simulink model "UZ_EnDat_be4_diffrework"  (R2023b)
settings: Solver=FixedStepDiscrete  StartTime=0  StopTime=0.002  RelTol=1e-3
model workspace (MAT data in the model file):
  Select = 0
libraries: hdlsllib x207, simulink x17, simulink_extras x3
(part 1 of 5)
settings Model: DataTypeOverride=Off  SimulationMode=accelerator  NumberOfSteps=10  PacingRate=1000  Creator=ELSYS_PC  LastModifiedBy=ELSYS_PC
settings SolverCC: AlgebraicLoopSolver=TrustRegion
settings DataIOCC: LimitDataPoints=on  SaveOutput=off  SaveTime=off
settings OptimizationCC: BlockReduction=off  ConditionallyExecuteInputs=off  DefaultParameterBehavior=Inlined  InheritOutputTypeSmallerThanSingle=on  LifeSpan=inf
settings DebuggingCC: AlgebraicLoopMsg=error  SingleTaskRateTransMsg=error  UnconnectedInputMsg=warning  UnconnectedOutputMsg=warning  UnconnectedLineMsg=warning  AllowSymbolicDim=off  StrictBusMsg=ErrorOnBusTreatedAsVector  SFUnexpectedBacktrackingDiag=warning  SFNoUnconditionalDefaultTransitionDiag=warning  SFExecutionAtInitializationDiag=none  ArithmeticOperatorsInVariantConditions=warning
settings HardwareCC: ProdBitPerPointer=32  ProdBitPerSizeT=32  ProdBitPerPtrDiffT=32  ProdLargestAtomicFloat=None  ProdIntDivRoundTo=Undefined  ProdEndianess=Unspecified  ProdWordSize=32  ProdHWDeviceType=ASIC/FPGA->ASIC/FPGA  TargetBitPerPointer=64  TargetBitPerSizeT=64  TargetBitPerPtrDiffT=64  TargetLongLongMode=on  TargetIntDivRoundTo=Zero  TargetEndianess=LittleEndian  TargetWordSize=64  TargetHWDeviceType=Custom Processor->MATLAB Host Computer  ProdEqTarget=off
settings ModelReferenceCC: EnableRefExpFcnMdlSchedulingChecks=on
settings SFSimCC: SimUseLocalCustomCode=off  CustomCodeUndefinedFunction=UseInterfaceOnly
settings RTWCC: RTWUseLocalCustomCode=off
settings CodeAppCC: StateflowObjectComments=on
settings GRTTargetCC: TargetLangStandard=C89/C90 (ANSI)  RTWCAPISignals=on  RTWCAPIParams=on
settings ConfigComp: CovScope=ReferencedModels  CovMetricSettings=dw  CovSaveCumulativeToWorkspaceVar=on  CovSaveSingleToWorkspaceVar=on  CovExternalEMLEnable=off  CovSFcnEnable=off  DVTestSuiteOptimization=Auto  DVDetectOutOfBounds=on  DVModelReferenceHarness=on  DVHarnessSource=Signal Editor  DVRebuildModelRepresentation=IfChangeIsDetected

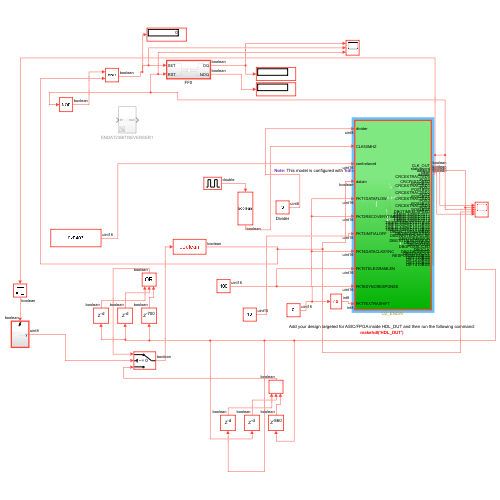
[thumbnail: Simulink's stored preview of the top-level diagram]
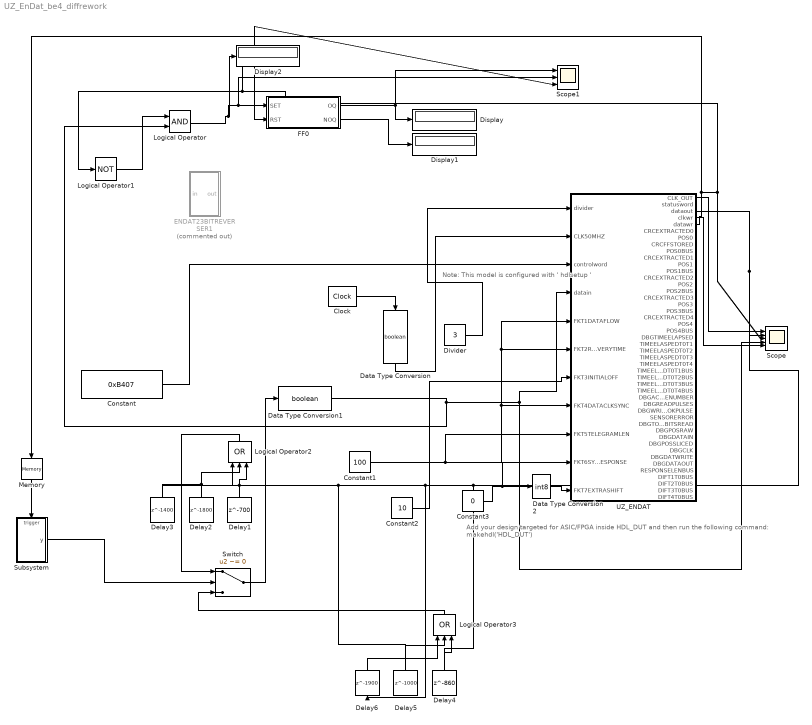
== system UZ_EnDat_be4_diffrework ==
  note: Note: This model is configured with ' hdlsetup '
  note: Add your design targeted for ASIC/FPGA inside HDL_DUT and then run the following command:
      | makehdl('HDL_DUT')
  Clock : simulink_extras/Flip Flops/Clock  period=2E-8
  Constant : Constant  Value=0xB407  OutDataTypeStr=uint16  SampleTime=-1
  Constant1 : Constant  Value=100  OutDataTypeStr=uint16  SampleTime=-1
  Constant2 : Constant  Value=10  OutDataTypeStr=uint16  SampleTime=-1
  Constant3 : Constant  Value=0  OutDataTypeStr=uint16  SampleTime=-1
  Data Type Conversion : DataTypeConversion  OutDataTypeStr=boolean  SaturateOnIntegerOverflow=off  RndMeth=Floor
  Data Type Conversion1 : DataTypeConversion  OutDataTypeStr=boolean  SaturateOnIntegerOverflow=off  RndMeth=Floor
  Data Type Conversion2 : DataTypeConversion  OutDataTypeStr=int8  SaturateOnIntegerOverflow=off  RndMeth=Floor
  Delay1 : Delay  DelayLength=700
  Delay2 : Delay  DelayLength=1800
  Delay3 : Delay  DelayLength=1400
  Delay4 : Delay  DelayLength=860
  Delay5 : Delay  DelayLength=1000
  Delay6 : Delay  DelayLength=1900
  Display : Display
  Display1 : Display
  Display2 : Display
  Divider : Constant  Value=3  OutMin=0  OutMax=7  OutDataTypeStr=uint8  SampleTime=-1
  ENDAT23BITREVERSER1 : Subsystem  Commented=on
  FF0 : Subsystem  TreatAsAtomicUnit=on
      settings: LibrarySourceBlock=|
      | hdlsllib/Ports &
      | Subsystems/Triggered
      | Subsystem
  Logical Operator : Logic  AllPortsSameDT=off  OutDataTypeStr=boolean
  Logical Operator1 : Logic  Operator=NOT  AllPortsSameDT=off  OutDataTypeStr=boolean
  Logical Operator2 : Logic  Operator=OR  Inputs=3  AllPortsSameDT=off  OutDataTypeStr=boolean
  Logical Operator3 : Logic  Operator=OR  Inputs=3  AllPortsSameDT=off  OutDataTypeStr=boolean
  Memory : Memory  InheritSampleTime=on
  Scope : Scope  NumInputPorts=5
  Scope1 : Scope  NumInputPorts=3
  Subsystem : Subsystem
  Switch : Switch  Criteria=u2 ~= 0  SaturateOnIntegerOverflow=off  InputSameDT=off
  UZ_ENDAT : Subsystem  TreatAsAtomicUnit=on
  wires:
  Constant/1 -> UZ_ENDAT/3(controlword)
  Data Type Conversion/1 -> UZ_ENDAT/2(CLK50MHZ)
  Divider/1 -> UZ_ENDAT/1(divider)
  Clock/1 -> Data Type Conversion/1
  Data Type Conversion1/1 -> Logical Operator/2, Scope/4, UZ_ENDAT/4(datain)
  Delay1/1 -> Logical Operator2/3
  UZ_ENDAT/1(CLK_OUT) -> Scope/1
  UZ_ENDAT/5(datawr) -> Memory/1, Scope1/3, FF0/2(RST), Logical Operator1/1, Scope/3
  Constant1/1 -> UZ_ENDAT/5(FKT1DATAFLOW), UZ_ENDAT/6(FKT2RECOVERYTIME), UZ_ENDAT/8(FKT4DATACLKSYNC), UZ_ENDAT/9(FKT5TELEGRAMLEN)
  Constant2/1 -> UZ_ENDAT/7(FKT3INITIALOFF)
  FF0/1(OQ) -> Scope1/1, Display/1
  Logical Operator/1 -> Scope1/2, FF0/1(SET), Display2/1
  FF0/2(NOQ) -> Display1/1
  Logical Operator1/1 -> Logical Operator/1
  Delay2/1 -> Logical Operator2/2
  Delay3/1 -> Logical Operator2/1
  Logical Operator2/1 -> Switch/1
  Switch/1 -> Data Type Conversion1/1
  Delay6/1 -> Logical Operator3/1
  Delay5/1 -> Logical Operator3/2
  Logical Operator3/1 -> Switch/3
  Delay4/1 -> Logical Operator3/3
  UZ_ENDAT/3(dataout) -> Delay4/1, Delay6/1, Delay3/1, Delay2/1, Delay1/1, Delay5/1, Scope/2
  Subsystem/1(y) -> Switch/2
  Memory/1 -> Subsystem/Trigger
  UZ_ENDAT/4(clkwr) -> Scope/5
  Constant3/1 -> UZ_ENDAT/10(FKT6SYNCRESPONSE), Data Type Conversion2/1
  Data Type Conversion2/1 -> UZ_ENDAT/11(FKT7EXTRASHIFT)

== system UZ_EnDat_be4_diffrework/ENDAT23BITREVERSER1 ==
  in : Inport
  16BITREVERSER : Subsystem
  16BITREVERSER1 : Subsystem
  Bit Concat : hdlsllib/Logic and Bit Operations/Bit Concat  numInputs=2
  Bit Shift : hdlsllib/Logic and Bit Operations/Bit Shift  mode=Shift Right Logical  N=8
  Bit Slice : hdlsllib/Logic and Bit Operations/Bit Slice  lidx=15  ridx=0
  Bit Slice1 : hdlsllib/Logic and Bit Operations/Bit Slice  lidx=22  ridx=16
  out : Outport
  wires:
  Bit Concat/1 -> Bit Shift/1
  Bit Shift/1 -> out/1
  in/1 -> Bit Slice1/1, Bit Slice/1
  Bit Slice/1 -> 16BITREVERSER/1(in)
  Bit Slice1/1 -> 16BITREVERSER1/1(in)
  16BITREVERSER/1(out) -> Bit Concat/1
  16BITREVERSER1/1(out) -> Bit Concat/2

== system UZ_EnDat_be4_diffrework/FF0 ==
  SET : Inport
  RST : Inport  Port=2
  S-R Flip-Flop : simulink_extras/Flip Flops/S-R Flip-Flop  initial_condition=0
  OQ : Outport
  NOQ : Outport  Port=2
  wires:
  SET/1 -> S-R Flip-Flop/1
  RST/1 -> S-R Flip-Flop/2
  S-R Flip-Flop/1 -> OQ/1
  S-R Flip-Flop/2 -> NOQ/1

== system UZ_EnDat_be4_diffrework/Subsystem ==
  Trigger : TriggerPort  VariantControl=(inherit)  PortDimensions=1
  Counter Limited : hdlsllib/Sources/Counter Limited  uplimit=1  tsamp=-1
  y : Outport
  wires:
  Counter Limited/1 -> y/1

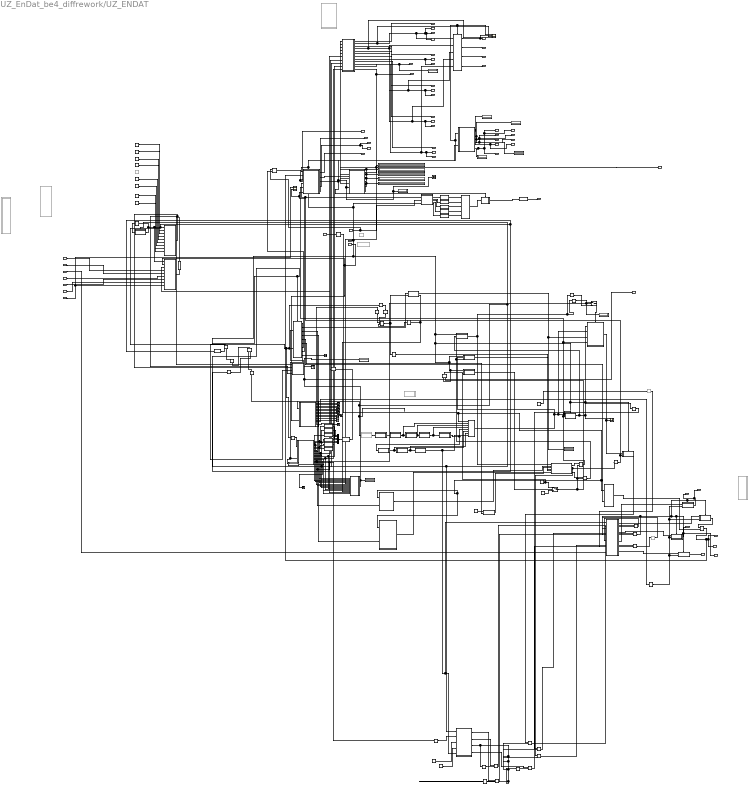
== system UZ_EnDat_be4_diffrework/UZ_ENDAT ==
  note: 0=12.5;1=6,25;2=3,125;3=1,5625
  divider : Inport  OutDataTypeStr=uint8  SampleTime=1e-8
  CLK50MHZ : Inport  Port=2  SampleTime=1e-8
  controlword : Inport  Port=3  OutDataTypeStr=uint16  SampleTime=1e-8
  datain : Inport  Port=4  OutDataTypeStr=boolean  SampleTime=1e-8
  FKT1DATAFLOW : Inport  Port=5  OutDataTypeStr=uint16  SampleTime=1e-8
  FKT2RECOVERYTIME : Inport  Port=6  OutDataTypeStr=uint16  SampleTime=1e-8
  FKT3INITIALOFF : Inport  Port=7  OutDataTypeStr=uint16  SampleTime=1e-8
  FKT4DATACLKSYNC : Inport  Port=8  OutDataTypeStr=uint16  SampleTime=1e-8
  FKT5TELEGRAMLEN : Inport  Port=9  OutDataTypeStr=uint16  SampleTime=1e-8
  FKT6SYNCRESPONSE : Inport  Port=10  OutDataTypeStr=uint16  SampleTime=1e-8
  FKT7EXTRASHIFT : Inport  Port=11  OutDataTypeStr=int8  SampleTime=1e-8
  16BIT_SPLITTER1 : Subsystem  Commented=on  TreatAsAtomicUnit=on
  16bitgather : Subsystem
      settings: LibrarySourceBlock=|
      | hdlsllib/Ports &
      | Subsystems/Subsystem
  2CLKDELAY : Delay  DelayLengthSource=Input port  DelayLength=10  DelayLengthUpperLimit=127  PreventDirectFeedthrough=on
      settings: InputPortMap=u0,p1
  5timestorage : Subsystem
      settings: LibrarySourceBlock=|
      | hdlsllib/Ports &
      | Subsystems/Subsystem
  8BIT_SPLITTER : Subsystem  TreatAsAtomicUnit=on
  8BIT_SPLITTER1 : Subsystem  TreatAsAtomicUnit=on
  Bits to Word : hdlsllib/Logic and Bit Operations/Bits to Word
  CLKCNTER_ACT : Subsystem
      settings: LibrarySourceBlock=|
      | hdlsllib/Ports &
      | Subsystems/Subsystem
  CLKCNTER_NOSTOP : Subsystem
      settings: LibrarySourceBlock=|
      | hdlsllib/Ports &
      | Subsystems/Subsystem
  CLKCNTER_RAMPUP : Subsystem
      settings: LibrarySourceBlock=|
      | hdlsllib/Ports &
      | Subsystems/Subsystem
  CLKDIV1 : Subsystem
  CLKDIV2 : Subsystem  Commented=through
  CLKDIV3 : Subsystem
  CLKDIV4 : Subsystem
  CLKDIV5 : Subsystem
  CLKDIV6 : Subsystem
  CLKDIV7 : Subsystem
  CLKDIV8 : Subsystem
  CLKDIV9 : Subsystem
  CONTROLWORDRAW : Subsystem
      settings: LibrarySourceBlock=|
      | hdlsllib/Ports &
      | Subsystems/Subsystem
  CONTROLWORDSTORED : Subsystem
      settings: LibrarySourceBlock=|
      | hdlsllib/Ports &
      | Subsystems/Subsystem
  CRC_Check : Subsystem  TreatAsAtomicUnit=on
  Compare To Constant : hdlsllib/Logic and Bit Operations/Compare To Constant  relop===  const=1  OutDataTypeStr=boolean
  Compare To Constant1 : hdlsllib/Logic and Bit Operations/Compare To Constant  relop===  const=1  OutDataTypeStr=boolean
  Compare To Constant2 : hdlsllib/Logic and Bit Operations/Compare To Constant  relop===  const=0  OutDataTypeStr=boolean
  Compare To Constant3 : hdlsllib/Logic and Bit Operations/Compare To Constant  relop=>=  const=3  OutDataTypeStr=boolean
  Compare To Constant4 : hdlsllib/Logic and Bit Operations/Compare To Constant  relop=>=  const=2  OutDataTypeStr=boolean
  Constant10 : Constant  Commented=on  Value=3  OutDataTypeStr=fixdt(0,4,0)  SampleTime=-1
  Constant11 : Constant  Commented=on  Value=0xB407  OutDataTypeStr=uint16  SampleTime=-1
  Constant12 : Constant  Value=48  OutDataTypeStr=uint16  SampleTime=-1
  Constant13 : Constant  Value=8  OutDataTypeStr=uint8  SampleTime=-1
  Constant3 : Constant  OutDataTypeStr=boolean  SampleTime=-1
  Constant6 : Constant  Value=51  OutDataTypeStr=uint16  SampleTime=-1
  ControlWordRAM : Constant  Value=0  VectorParams1D=off  OutDataTypeStr=uint8  SampleTime=-1
  DATA2CLOCKSYNCER : Subsystem
  DATA2CLOCKSYNCER1 : Subsystem  Commented=on
  DATAFLOWCHGER : Subsystem
  Data Type Conversion : DataTypeConversion  OutDataTypeStr=fixdt(0,4,0)  RndMeth=Nearest
  Data Type Conversion1 : DataTypeConversion  OutDataTypeStr=uint8  SaturateOnIntegerOverflow=off  RndMeth=Floor
  Data Type Conversion{2..12} (11 alike) : DataTypeConversion  OutMax=1  OutDataTypeStr=fixdt(0,1)  SaturateOnIntegerOverflow=off  RndMeth=Floor
  Delay : Delay  DelayLength=10  InitialCondition=0
  Delay1 : Delay  DelayLengthSource=Input port  DelayLengthUpperLimit=127  InitialCondition=0
      settings: InputPortMap=u0,p1
  Delay2 : Delay  DelayLength=1
  Delay3 : Delay  DelayLength=1
  Delay4 : Delay  DelayLength=0
  Detect Change : simulink/Logic and Bit Operations/Detect Change  vinit=0  OutDataTypeStr=boolean
      settings: LibrarySourceBlock=|
      | hdlsllib/Logic and Bit
      | Operations/Detect
      | Change
  Display{,1..15} (16 alike) : Display
      Display settings: Format=hex (Stored Integer)
      Display1 settings: Format=binary (Stored Integer)
      Display2 settings: Format=binary (Stored Integer)
      Display3 settings: Format=binary (Stored Integer)
      Display4 settings: Format=binary (Stored Integer)
      Display5 settings: Format=binary (Stored Integer)
      Display7 settings: Format=hex (Stored Integer)
      Display8 settings: Format=hex (Stored Integer)
      Display9 settings: Format=hex (Stored Integer)
  Dual Port RAM System : hdlsllib/HDL RAMs/Dual Port RAM System  RAMType=Dual port  AsyncRead=off  WriteOutputValue=New data  RAMInitialValue=0  allowBusInputs=off  WritesHaveOutput=on  NumReads=0  NumWrites=1  SimulateUsing=Code generation
  EndatControlRAM : Constant  VectorParams1D=off  OutDataTypeStr=uint8  SampleTime=-1
  FKT1 : Constant  Value=2  VectorParams1D=off  OutDataTypeStr=uint8  SampleTime=-1
  FKT2 : Constant  Value=3  VectorParams1D=off  OutDataTypeStr=uint8  SampleTime=-1
  FKT3 : Constant  Commented=on  Value=4  VectorParams1D=off  OutDataTypeStr=uint8  SampleTime=-1
  FKT4 : Constant  Value=5  VectorParams1D=off  OutDataTypeStr=uint8  SampleTime=-1
  FKT5 : Constant  Value=6  VectorParams1D=off  OutDataTypeStr=uint8  SampleTime=-1
  FKT6 : Constant  Value=7  VectorParams1D=off  OutDataTypeStr=uint8  SampleTime=-1
  FKT7 : Constant  Value=8  VectorParams1D=off  OutDataTypeStr=uint8  SampleTime=-1
  INITIALOFF : Subsystem
  Logical Operator{,1,7,9,13..14,16,18,20} (9 alike) : Logic  AllPortsSameDT=off  OutDataTypeStr=boolean
  Logical Operator10 : Logic  Operator=NOT  Inputs=3  AllPortsSameDT=off  OutDataTypeStr=boolean
  Logical Operator{5,11,15,22..23} (5 alike) : Logic  Operator=OR  AllPortsSameDT=off  OutDataTypeStr=boolean
  Logical Operator{2..4,17,19,21,24,27} (8 alike) : Logic  Operator=NOT  AllPortsSameDT=off  OutDataTypeStr=boolean
  Logical Operator25 : Logic  Commented=through  Operator=NOT  AllPortsSameDT=off  OutDataTypeStr=boolean
  Logical Operator26 : Logic  Commented=through  Operator=NOT  AllPortsSameDT=off  OutDataTypeStr=boolean
  Logical Operator6 : Logic  Operator=NOT  Inputs=3  AllPortsSameDT=off  OutDataTypeStr=boolean
  Logical Operator8 : Logic  Inputs=3  AllPortsSameDT=off  OutDataTypeStr=boolean
  ManualSerialize : Subsystem
      settings: LibrarySourceBlock=|
      | hdlsllib/Ports &
      | Subsystems/Subsystem
  Memory : Memory  InheritSampleTime=on
  Multiport Switch : MultiPortSwitch  DataPortOrder=Zero-based contiguous  Inputs=7  DataPortIndices={8,16,32,64}  zeroidx=on  SaturateOnIntegerOverflow=off  InputSameDT=off
  OUTPUTCONTROLCONTINIOUS : Subsystem
      settings: LibrarySourceBlock=|
      | hdlsllib/Ports &
      | Subsystems/Subsystem
  RAM_SELECTOR : MultiPortSwitch  DataPortOrder=Zero-based contiguous  Inputs=8  DataPortForDefault=Additional data port  zeroidx=on  OutDataTypeStr=uint8  SaturateOnIntegerOverflow=off  InputSameDT=off
  RAM_SELECTOR1 : MultiPortSwitch  DataPortOrder=Zero-based contiguous  Inputs=8  DataPortForDefault=Additional data port  zeroidx=on  SaturateOnIntegerOverflow=off  InputSameDT=off
  RAM_SELECTOR2 : MultiPortSwitch  Commented=on  DataPortOrder=Zero-based contiguous  Inputs=16  DataPortForDefault=Additional data port  zeroidx=on  SaturateOnIntegerOverflow=off  InputSameDT=off
  RECOVERYTIMESELECTOR : Subsystem
  RESPONSESLICER5X : Subsystem
  Scope : Scope
  Scope1 : Scope  NumInputPorts=2
  Scope2 : Scope  NumInputPorts=2
  Scope3 : Scope  NumInputPorts=4
  SetZero32modified : Subsystem  Commented=on
  SetZeroBool : Subsystem
  SetZeroBool1 : Subsystem
  SetZeroBool2 : Subsystem
  SetZeroBool3 : Subsystem
  SetZeroBool4 : Subsystem
  SetZeroBool5 : Subsystem
  Signal Specification : SignalSpecification  OutDataTypeStr=uint16
  Storage16 : Subsystem
      settings: LibrarySourceBlock=|
      | hdlsllib/Ports &
      | Subsystems/Subsystem
  Subsystem : Subsystem
  Subsystem1 : Subsystem
  Subsystem2 : Subsystem
  Subsystem6 : Subsystem
  Switch : Switch  Criteria=u2 > Threshold  SaturateOnIntegerOverflow=off  InputSameDT=off
  Terminator{,1,4,12..17,19..25} (16 alike) : Terminator
  Vector Concatenate : Concatenate  NumInputs=6
  Vector Concatenate1 : Concatenate  NumInputs=5
  deadtime : Switch  Threshold=2000  SaturateOnIntegerOverflow=off  InputSameDT=off
  deadtimeconst1 : Constant  OutDataTypeStr=boolean  SampleTime=-1
  deadtimeconst2 : Constant  Value=0  OutDataTypeStr=boolean  SampleTime=-1
  ramselektor : Subsystem  TreatAsAtomicUnit=on
      settings: LibrarySourceBlock=|
      | hdlsllib/Ports &
      | Subsystems/Triggered
      | Subsystem
  responseslicer5 : Subsystem  Commented=on  TreatAsAtomicUnit=on
      settings: LibrarySourceBlock=|
      | hdlsllib/Ports &
      | Subsystems/Subsystem
  timingprovider : Subsystem
      settings: LibrarySourceBlock=|
      | hdlsllib/Ports &
      | Subsystems/Subsystem
  CLK_OUT : Outport  VectorParamsAs1DForOutWhenUnconnected=off
  statusword : Outport  Port=2  OutDataTypeStr=uint16  VectorParamsAs1DForOutWhenUnconnected=off
  dataout : Outport  Port=3  OutDataTypeStr=boolean  VectorParamsAs1DForOutWhenUnconnected=off
  clkwr : Outport  Port=4  OutDataTypeStr=boolean  VectorParamsAs1DForOutWhenUnconnected=off
  datawr : Outport  Port=5  OutDataTypeStr=boolean  VectorParamsAs1DForOutWhenUnconnected=off
  CRCEXTRACTED0 : Outport  Port=6  OutDataTypeStr=uint8  VectorParamsAs1DForOutWhenUnconnected=off
  POS0 : Outport  Port=7  OutDataTypeStr=uint32  VectorParamsAs1DForOutWhenUnconnected=off
  CRCFFSTORED : Outport  Port=8  OutDataTypeStr=uint8  VectorParamsAs1DForOutWhenUnconnected=off
  POS0BUS : Outport  Port=9  OutDataTypeStr=uint32  VectorParamsAs1DForOutWhenUnconnected=off
  CRCEXTRACTED1 : Outport  Port=10  OutDataTypeStr=uint8  VectorParamsAs1DForOutWhenUnconnected=off
  POS1 : Outport  Port=11  OutDataTypeStr=uint32  VectorParamsAs1DForOutWhenUnconnected=off
  POS1BUS : Outport  Port=12  OutDataTypeStr=uint32  VectorParamsAs1DForOutWhenUnconnected=off
  CRCEXTRACTED2 : Outport  Port=13  OutDataTypeStr=uint8  VectorParamsAs1DForOutWhenUnconnected=off
  POS2 : Outport  Port=14  OutDataTypeStr=uint32  VectorParamsAs1DForOutWhenUnconnected=off
  POS2BUS : Outport  Port=15  OutDataTypeStr=uint32  VectorParamsAs1DForOutWhenUnconnected=off
  CRCEXTRACTED3 : Outport  Port=16  OutDataTypeStr=uint8  VectorParamsAs1DForOutWhenUnconnected=off
  POS3 : Outport  Port=17  OutDataTypeStr=uint32  VectorParamsAs1DForOutWhenUnconnected=off
  POS3BUS : Outport  Port=18  OutDataTypeStr=uint32  VectorParamsAs1DForOutWhenUnconnected=off
  CRCEXTRACTED4 : Outport  Port=19  OutDataTypeStr=uint8  VectorParamsAs1DForOutWhenUnconnected=off
  POS4 : Outport  Port=20  OutDataTypeStr=uint32  VectorParamsAs1DForOutWhenUnconnected=off
  POS4BUS : Outport  Port=21  OutDataTypeStr=uint32  VectorParamsAs1DForOutWhenUnconnected=off
  DBGTIMEELAPSED : Outport  Port=22  VectorParamsAs1DForOutWhenUnconnected=off
  TIMEELASPEDT0T1 : Outport  Port=23  VectorParamsAs1DForOutWhenUnconnected=off
  TIMEELASPEDT0T2 : Outport  Port=24  VectorParamsAs1DForOutWhenUnconnected=off
  TIMEELASPEDT0T3 : Outport  Port=25  VectorParamsAs1DForOutWhenUnconnected=off
  TIMEELASPEDT0T4 : Outport  Port=26  VectorParamsAs1DForOutWhenUnconnected=off
  TIMEELASPEDT0T1BUS : Outport  Port=27  VectorParamsAs1DForOutWhenUnconnected=off
  TIMEELASPEDT0T2BUS : Outport  Port=28  VectorParamsAs1DForOutWhenUnconnected=off
  TIMEELASPEDT0T3BUS : Outport  Port=29  VectorParamsAs1DForOutWhenUnconnected=off
  TIMEELASPEDT0T4BUS : Outport  Port=30  VectorParamsAs1DForOutWhenUnconnected=off
  DBGACTIVENUMBER : Outport  Port=31  OutDataTypeStr=uint8  VectorParamsAs1DForOutWhenUnconnected=off
  DBGREADPULSES : Outport  Port=32  OutDataTypeStr=boolean  VectorParamsAs1DForOutWhenUnconnected=off
  DBGWRITEOKPULSE : Outport  Port=33  OutDataTypeStr=boolean  VectorParamsAs1DForOutWhenUnconnected=off
  SENSORERROR : Outport  Port=34  OutDataTypeStr=boolean  VectorParamsAs1DForOutWhenUnconnected=off
  DBGTOTALBITSREAD : Outport  Port=35  VectorParamsAs1DForOutWhenUnconnected=off
  DBGPOSRAW : Outport  Port=36  OutDataTypeStr=uint64  VectorParamsAs1DForOutWhenUnconnected=off
  DBGDATAIN : Outport  Port=37  OutDataTypeStr=boolean  VectorParamsAs1DForOutWhenUnconnected=off
  DBGPOSSLICED : Outport  Port=38  OutDataTypeStr=uint32  VectorParamsAs1DForOutWhenUnconnected=off
  DBGCLK : Outport  Port=39  VectorParamsAs1DForOutWhenUnconnected=off
  DBGDATWRITE : Outport  Port=40  VectorParamsAs1DForOutWhenUnconnected=off
  DBGDATAOUT : Outport  Port=41  OutDataTypeStr=boolean  VectorParamsAs1DForOutWhenUnconnected=off
  RESPONSELENBUS : Outport  Port=42  VectorParamsAs1DForOutWhenUnconnected=off
  DIFT1T0BUS : Outport  Port=43  OutDataTypeStr=int32  VectorParamsAs1DForOutWhenUnconnected=off
  DIFT2T0BUS : Outport  Port=44  OutDataTypeStr=int32  VectorParamsAs1DForOutWhenUnconnected=off
  DIFT3T0BUS : Outport  Port=45  OutDataTypeStr=int32  VectorParamsAs1DForOutWhenUnconnected=off
  DIFT4T0BUS : Outport  Port=46  OutDataTypeStr=int32  VectorParamsAs1DForOutWhenUnconnected=off
  wires:
  CLKDIV2/1(CLK/2) -> CLKDIV1/1(CLK1)
  CLKDIV1/1(CLK/2) -> CLKDIV3/1(CLK1)
  CLKDIV3/1(CLK/2) -> CLKDIV4/1(CLK1), Multiport Switch/2
  CLKDIV4/1(CLK/2) -> CLKDIV5/1(CLK1), Multiport Switch/3
  CLKDIV5/1(CLK/2) -> CLKDIV6/1(CLK1), Multiport Switch/4
  CLKDIV6/1(CLK/2) -> CLKDIV7/1(CLK1), Multiport Switch/5
  controlword/1 -> CONTROLWORDRAW/2(DATA), RAM_SELECTOR1/2
  Dual Port RAM System/1 -> Terminator1/1
  RAM_SELECTOR/1 -> Dual Port RAM System/2, Dual Port RAM System/4
  ControlWordRAM/1 -> RAM_SELECTOR/2
  Dual Port RAM System/2 -> 8BIT_SPLITTER/1(DATAIN)
  Memory/1 -> ramselektor/1(In1)
  RAM_SELECTOR1/1 -> Signal Specification/1
  Signal Specification/1 -> Dual Port RAM System/1
  EndatControlRAM/1 -> RAM_SELECTOR/3
  Delay/1 -> RAM_SELECTOR1/3
  Detect Change/1 -> Logical Operator/1
  Logical Operator2/1 -> Logical Operator/2
  Compare To Constant/1 -> Logical Operator1/2
  Logical Operator3/1 -> Logical Operator1/1
  Logical Operator1/1 -> Logical Operator2/1
  Logical Operator/1 -> Dual Port RAM System/3
  8BIT_SPLITTER/2(DATAOUT1) -> Storage16/1(Data)
  datain/1 -> Delay1/1, CRC_Check/2(data)
  CLKDIV7/1(CLK/2) -> CLKDIV8/1(CLK1), Multiport Switch/6
  CLKDIV8/1(CLK/2) -> CLKDIV9/1(CLK1), Multiport Switch/7
  CLKDIV9/1(CLK/2) -> Multiport Switch/8, Subsystem/5(VERYSLOWCLK), INITIALOFF/1(CLKAUX)
  Constant3/1 -> Logical Operator25/1
  CLKCNTER_ACT/1(CNT) -> Compare To Constant4/1, Compare To Constant3/1, OUTPUTCONTROLCONTINIOUS/1(CLKCNT)
  Subsystem6/1(Out1) -> OUTPUTCONTROLCONTINIOUS/3(CLK2ENDOFTRANSMISSION)
  OUTPUTCONTROLCONTINIOUS/2(DATAINV) -> Logical Operator4/1, Logical Operator14/1
  Logical Operator4/1 -> ManualSerialize/4(recieving), CRC_Check/1(set), SetZeroBool1/2(setzero)
  Storage16/2(wrok) -> Logical Operator6/1, 16bitgather/14(wrok)
  ramselektor/1(SEL) -> RAM_SELECTOR1/1, RAM_SELECTOR/1, Compare To Constant/1, Detect Change/1, Compare To Constant2/1, Compare To Constant1/1, 8BIT_SPLITTER/2(SEL), Memory/1
  Compare To Constant1/1 -> Delay3/1
  Logical Operator6/1 -> Logical Operator8/3
  Delay2/1 -> Logical Operator8/1
  Delay3/1 -> Logical Operator8/2
  Logical Operator8/1 -> Logical Operator10/1, Storage16/2(Write)
  Logical Operator10/1 -> OUTPUTCONTROLCONTINIOUS/4(OPENCOM)
  Logical Operator5/1 -> CLKCNTER_NOSTOP/3(ResetCNT), CLKCNTER_ACT/3(ResetCNT)
  Storage16/1(out) -> Subsystem2/3(DATA), Display/1
  SetZeroBool/1(valueout) -> CLKCNTER_ACT/2(CLK2CNT), Delay4/1, Scope1/1
  Delay4/1 -> Logical Operator13/1
  OUTPUTCONTROLCONTINIOUS/1(CLKOFF) -> Logical Operator11/1
  deadtime/1 -> Logical Operator5/2, Logical Operator11/2, Logical Operator7/2
  OUTPUTCONTROLCONTINIOUS/3(RESETCNT) -> Logical Operator5/1
  CLKCNTER_RAMPUP/1(CNT) -> deadtime/2
  deadtimeconst2/1 -> CLKCNTER_RAMPUP/3(ResetCNT), deadtime/1
  deadtimeconst1/1 -> deadtime/3
  Logical Operator7/1 -> CLKCNTER_RAMPUP/2(CLK2CNT)
  Subsystem2/1(valin) -> SetZeroBool1/1(valin), Scope1/2
  CONTROLWORDRAW/14(DATAOUT13) -> Delay2/1
  CONTROLWORDSTORED/7(DATAOUT6) -> 16bitgather/7(DATAOUT7), Display15/1, Switch/2
  CONTROLWORDRAW/16(DATAOUT15) -> Logical Operator3/1
  Compare To Constant2/1 -> CONTROLWORDSTORED/1(CLK)
  CONTROLWORDSTORED/1(DATAOUT0) -> 16bitgather/1(in1), Data Type Conversion4/1
  CONTROLWORDSTORED/3(DATAOUT2) -> Data Type Conversion6/1, 16bitgather/3(DATAOUT3)
  CONTROLWORDSTORED/4(DATAOUT3) -> 16bitgather/4(DATAOUT4), Data Type Conversion7/1
  CONTROLWORDSTORED/5(DATAOUT4) -> 16bitgather/5(DATAOUT5), Data Type Conversion8/1
  CONTROLWORDSTORED/6(DATAOUT5) -> Data Type Conversion9/1
  Vector Concatenate/1 -> Bits to Word/1
  Data Type Conversion4/1 -> Vector Concatenate/1
  CONTROLWORDSTORED/2(DATAOUT1) -> 16bitgather/2(DATAOUT1), Data Type Conversion5/1
  Data Type Conversion5/1 -> Vector Concatenate/2
  Data Type Conversion6/1 -> Vector Concatenate/3
  Data Type Conversion7/1 -> Vector Concatenate/4
  Data Type Conversion8/1 -> Vector Concatenate/5
  Data Type Conversion9/1 -> Vector Concatenate/6
  Bits to Word/1 -> Delay/1
  CONTROLWORDSTORED/15(DATAOUT14) -> 16bitgather/15(DATAOUT14), Logical Operator24/1
  Data Type Conversion/1 -> Multiport Switch/1, DATA2CLOCKSYNCER/1(In1), DATAFLOWCHGER/1(CLKSEL), RECOVERYTIMESELECTOR/1(In1)
  5timestorage/1(t0) -> Display1/1, DBGPOSRAW/1, RESPONSESLICER5X/1(DATA)
  Logical Operator9/1 -> Logical Operator23/2
  Logical Operator13/1 -> Logical Operator22/1
  Logical Operator14/1 -> Logical Operator15/1
  Logical Operator15/1 -> Logical Operator26/1
  Logical Operator17/1 -> Logical Operator16/2
  Logical Operator19/1 -> Logical Operator18/2
  Logical Operator21/1 -> Logical Operator20/2
  Logical Operator16/1 -> Logical Operator15/2
  Logical Operator18/1 -> Logical Operator22/2
  Logical Operator20/1 -> Logical Operator23/1
  Logical Operator25/1 -> INITIALOFF/5(CLKWR)
  Logical Operator23/1 -> INITIALOFF/4(DATA)
  CLK50MHZ/1 -> timingprovider/2(clk), ManualSerialize/1(CLK), CRC_Check/3(clk), CLKCNTER_NOSTOP/1(CLK), CLKCNTER_RAMPUP/1(CLK), Logical Operator7/1, Subsystem2/1(CLK), SetZeroBool1/Trigger, CLKCNTER_ACT/1(CLK), Subsystem/1(CLK), CLKDIV2/1(CLK1), CONTROLWORDRAW/1(CLK), ramselektor/Trigger, 8BIT_SPLITTER/Trigger
  SetZeroBool5/1(valueout) -> 2CLKDELAY/1
  Logical Operator26/1 -> INITIALOFF/3(DATAWR)
  Logical Operator22/1 -> INITIALOFF/2(CLK), SetZeroBool2/Trigger, SetZeroBool4/Trigger, SetZeroBool5/Trigger, SetZeroBool3/Trigger
  Multiport Switch/1 -> CLKCNTER_NOSTOP/2(CLK2CNT), Subsystem2/2(SLOWCLCK), SetZeroBool/Trigger, SetZeroBool/1(valin)
  SetZeroBool4/1(valueout) -> datawr/1, DBGDATWRITE/1
  INITIALOFF/3(DATA_OUT) -> SetZeroBool3/1(valin)
  SetZeroBool2/1(valueout) -> clkwr/1
  8BIT_SPLITTER/1(DATAOUT0) -> Display7/1, CONTROLWORDSTORED/2(DATA)
  SetZeroBool1/1(valueout) -> Logical Operator9/1
  DATAFLOWCHGER/1(Output) -> OUTPUTCONTROLCONTINIOUS/2(CLKS2DATAFLOWCHG)
  FKT1DATAFLOW/1 -> RAM_SELECTOR1/4
  CRC_Check/2(CRC1) -> Data Type Conversion2/1
  CRC_Check/3(CRC2) -> Data Type Conversion3/1
  CRC_Check/4(CRC3) -> Data Type Conversion10/1
  CRC_Check/5(CRC4) -> Data Type Conversion11/1
  CRC_Check/6(CRC5) -> Data Type Conversion12/1
  RECOVERYTIMESELECTOR/1(Out1) -> OUTPUTCONTROLCONTINIOUS/6(RECOVERYTIME)
  DATA2CLOCKSYNCER/1(Out1) -> 2CLKDELAY/2
  Constant6/1 -> Subsystem6/1(In1)
  Data Type Conversion2/1 -> Vector Concatenate1/1
  Data Type Conversion3/1 -> Vector Concatenate1/2
  Data Type Conversion10/1 -> Vector Concatenate1/3
  Data Type Conversion11/1 -> Vector Concatenate1/4
  Data Type Conversion12/1 -> Vector Concatenate1/5
  Vector Concatenate1/1 -> Subsystem1/1(in)
  Subsystem1/1(out) -> Data Type Conversion1/1
  5timestorage/2(t-1) -> Display2/1, RESPONSESLICER5X/2(DATA1)
  5timestorage/3(t-2) -> Display3/1, RESPONSESLICER5X/3(DATA2)
  5timestorage/4(t-3) -> Display4/1, RESPONSESLICER5X/4(DATA3)
  5timestorage/5(t-4) -> Display5/1, RESPONSESLICER5X/5(DATA4)
  FKT1/1 -> RAM_SELECTOR/4
  FKT2/1 -> RAM_SELECTOR/5
  FKT4/1 -> RAM_SELECTOR/6
  FKT5/1 -> RAM_SELECTOR/7
  FKT2RECOVERYTIME/1 -> RAM_SELECTOR1/5
  FKT4DATACLKSYNC/1 -> RAM_SELECTOR1/6
  FKT5TELEGRAMLEN/1 -> RAM_SELECTOR1/7
  8BIT_SPLITTER/3(DATAOUT2) -> DATAFLOWCHGER/2(FACTOR)
  8BIT_SPLITTER/4(DATAOUT3) -> RECOVERYTIMESELECTOR/2(FAKTOR)
  8BIT_SPLITTER/5(DATAOUT4) -> DATA2CLOCKSYNCER/2(FAKTOR)
  8BIT_SPLITTER/6(DATAOUT5) -> Subsystem6/2(FACTOR)
  divider/1 -> Data Type Conversion/1
  Data Type Conversion1/1 -> CRCFFSTORED/1
  timingprovider/4(timeelapsed1cycl) -> Display11/1, DBGTIMEELAPSED/1, TIMEELASPEDT0T1/1, TIMEELASPEDT0T1BUS/1
  timingprovider/3(timeelapsed2cycl) -> TIMEELASPEDT0T2/1, TIMEELASPEDT0T2BUS/1, Display14/1
  timingprovider/2(timeelapsed3cycl) -> Display13/1, TIMEELASPEDT0T3BUS/1, TIMEELASPEDT0T3/1
  timingprovider/1(timeelapsed4cycl) -> TIMEELASPEDT0T4BUS/1, TIMEELASPEDT0T4/1, Display12/1
  RESPONSESLICER5X/8(payload3) -> 8BIT_SPLITTER1/4(DATAT3), POS3BUS/1, POS3/1
  RESPONSESLICER5X/6(payload2) -> 8BIT_SPLITTER1/3(DATAT2), POS2BUS/1, POS2/1
  RESPONSESLICER5X/10(payload4) -> 8BIT_SPLITTER1/5(DATAT4), POS4BUS/1, POS4/1
  RESPONSESLICER5X/4(payload1) -> Scope3/4, 8BIT_SPLITTER1/2(DATAT1), POS1BUS/1, POS1/1
  RESPONSESLICER5X/2(payload) -> Scope3/3, 8BIT_SPLITTER1/1(DATAT0), POS0/1, DBGPOSSLICED/1, POS0BUS/1
  RESPONSESLICER5X/1(CRC) -> CRCEXTRACTED0/1
  RESPONSESLICER5X/3(CRC1) -> CRCEXTRACTED1/1
  RESPONSESLICER5X/5(CRC2) -> CRCEXTRACTED2/1
  RESPONSESLICER5X/7(CRC3) -> CRCEXTRACTED3/1
  RESPONSESLICER5X/9(CRC4) -> CRCEXTRACTED4/1
  CONTROLWORDSTORED/8(DATAOUT7) -> RESPONSESLICER5X/6(19BIT), 16bitgather/8(DATAOUT8)
  CONTROLWORDSTORED/9(DATAOUT8) -> RESPONSESLICER5X/7(21BIT), 16bitgather/9(DATAOUT9)
  CONTROLWORDSTORED/10(DATAOUT9) -> RESPONSESLICER5X/8(23BIT), 16bitgather/10(DATAOUT10)
  CONTROLWORDSTORED/11(DATAOUT10) -> RESPONSESLICER5X/9(25BIT), 16bitgather/11(In11)
  CONTROLWORDSTORED/12(DATAOUT11) -> RESPONSESLICER5X/10(27BIT), 16bitgather/12(DATAOUT11)
  CONTROLWORDSTORED/13(DATAOUT12) -> 16bitgather/13(DATAOUT12)
  CONTROLWORDSTORED/16(DATAOUT15) -> 16bitgather/16(DATAOUT15)
  INITIALOFF/4(CLKWR_OUT) -> SetZeroBool2/1(valin)
  SetZeroBool3/1(valueout) -> DBGDATAOUT/1, dataout/1
  Logical Operator27/1 -> SetZeroBool5/2(setzero), SetZeroBool3/2(setzero), SetZeroBool4/2(setzero), SetZeroBool2/2(setzero)
  INITIALOFF/2(DATAWR_OUT) -> SetZeroBool4/1(valin)
  INITIALOFF/1(CLK_OUT) -> SetZeroBool5/1(valin)
  RESPONSESLICER5X/11(DBGACTIVENUMBER) -> DBGACTIVENUMBER/1, Display10/1
  ManualSerialize/3(wrok) -> Subsystem1/Enable, Scope/1, Display6/1, 5timestorage/2(wrok), Scope3/1, 8BIT_SPLITTER1/Trigger, timingprovider/1(wrok)
  ManualSerialize/2(valueout) -> 5timestorage/1(DATA)
  CLKCNTER_NOSTOP/1(CNT) -> OUTPUTCONTROLCONTINIOUS/5(CLKCNTNOSTOP)
  ManualSerialize/1(dbg) -> DBGREADPULSES/1
  ManualSerialize/5(dbg1) -> DBGWRITEOKPULSE/1
  ManualSerialize/4(dbg2) -> RESPONSELENBUS/1, DBGTOTALBITSREAD/1
  RESPONSESLICER5X/12(sensorerror) -> 16bitgather/6(DATAOUT6), SENSORERROR/1
  16bitgather/1(statusword) -> statusword/1, Display8/1, Display9/1
  Subsystem/3(BOOTUPCOMPLETE) -> Logical Operator17/1, Logical Operator19/1, Logical Operator14/2, Logical Operator13/2, Logical Operator9/2, Logical Operator21/1
  Logical Operator24/1 -> Subsystem/2(RESET)
  Constant13/1 -> Subsystem/3(CLKS2DATAFLOWCHG)
  Constant12/1 -> Subsystem/4(CLK2ENDOFTRANSMISSION)
  Subsystem/1(CLKOUT) -> Logical Operator18/1
  Subsystem/2(DATAOUT) -> Logical Operator20/1
  Subsystem/4(DATAINV) -> Logical Operator16/1
  CONTROLWORDSTORED/14(DATAOUT13) -> Terminator/1
  8BIT_SPLITTER/7(DATAOUT6) -> Delay1/2
  8BIT_SPLITTER/8(DATAOUT7) -> Scope2/2, ManualSerialize/6(FKT7EXTRASHIFTER)
  8BIT_SPLITTER/9(DATAOUT8) -> Terminator4/1
  CONTROLWORDRAW/1(DATAOUT0) -> Terminator12/1
  CONTROLWORDRAW/2(DATAOUT1) -> Terminator13/1
  CONTROLWORDRAW/3(DATAOUT2) -> Terminator14/1
  CONTROLWORDRAW/4(DATAOUT3) -> Terminator15/1
  CONTROLWORDRAW/5(DATAOUT4) -> Terminator16/1
  CONTROLWORDRAW/15(DATAOUT14) -> Terminator17/1
  CONTROLWORDRAW/12(DATAOUT11) -> Terminator19/1
  CONTROLWORDRAW/11(DATAOUT10) -> Terminator20/1
  CONTROLWORDRAW/10(DATAOUT9) -> Terminator21/1
  CONTROLWORDRAW/6(DATAOUT5) -> Terminator22/1
  CONTROLWORDRAW/7(DATAOUT6) -> Terminator23/1
  CONTROLWORDRAW/8(DATAOUT7) -> Terminator24/1
  CONTROLWORDRAW/9(DATAOUT8) -> Terminator25/1
  Compare To Constant3/1 -> Switch/3
  Compare To Constant4/1 -> Switch/1
  Switch/1 -> Subsystem2/Enable
  2CLKDELAY/1 -> ManualSerialize/2(SLOWCLCK), CLK_OUT/1, DBGCLK/1
  FKT3INITIALOFF/1 -> INITIALOFF/6(FACTOR)
  CONTROLWORDRAW/13(DATAOUT12) -> Logical Operator27/1
  Logical Operator11/1 -> ManualSerialize/5(clkoff), Subsystem2/4(reset), SetZeroBool/2(setzero)
  Delay1/1 -> DBGDATAIN/1, ManualSerialize/3(DATA)
  FKT6SYNCRESPONSE/1 -> RAM_SELECTOR1/8
  FKT7EXTRASHIFT/1 -> Scope2/1, RAM_SELECTOR1/9
  FKT6/1 -> RAM_SELECTOR/8
  FKT7/1 -> RAM_SELECTOR/9
  8BIT_SPLITTER1/1(DIFT1T0) -> Scope3/2, DIFT1T0BUS/1
  8BIT_SPLITTER1/2(DIFT2T0) -> DIFT2T0BUS/1
  8BIT_SPLITTER1/3(DIFT3T0) -> DIFT3T0BUS/1
  8BIT_SPLITTER1/4(DIFT4T0) -> DIFT4T0BUS/1

== system UZ_EnDat_be4_diffrework/ENDAT23BITREVERSER1/16BITREVERSER ==
  in : Inport
  Bit Concat : hdlsllib/Logic and Bit Operations/Bit Concat  numInputs=4
  Bit Slice : hdlsllib/Logic and Bit Operations/Bit Slice  lidx=3  ridx=0
  Bit Slice1 : hdlsllib/Logic and Bit Operations/Bit Slice  lidx=7  ridx=4
  Bit Slice2 : hdlsllib/Logic and Bit Operations/Bit Slice  lidx=11  ridx=8
  Bit Slice3 : hdlsllib/Logic and Bit Operations/Bit Slice  lidx=15  ridx=12
  out : Outport
  wires:
  in/1 -> Bit Slice/1, Bit Slice3/1, Bit Slice2/1, Bit Slice1/1
  Bit Slice1/1 -> Bit Concat/2
  Bit Slice/1 -> Bit Concat/1
  Bit Slice2/1 -> Bit Concat/3
  Bit Slice3/1 -> Bit Concat/4
  Bit Concat/1 -> out/1

== system UZ_EnDat_be4_diffrework/ENDAT23BITREVERSER1/16BITREVERSER1 ==
  in : Inport
  Bit Concat : hdlsllib/Logic and Bit Operations/Bit Concat  numInputs=4
  Bit Slice : hdlsllib/Logic and Bit Operations/Bit Slice  lidx=3  ridx=0
  Bit Slice1 : hdlsllib/Logic and Bit Operations/Bit Slice  lidx=7  ridx=4
  Bit Slice2 : hdlsllib/Logic and Bit Operations/Bit Slice  lidx=11  ridx=8
  Bit Slice3 : hdlsllib/Logic and Bit Operations/Bit Slice  lidx=15  ridx=12
  out : Outport
  wires:
  in/1 -> Bit Slice/1, Bit Slice3/1, Bit Slice2/1, Bit Slice1/1
  Bit Slice1/1 -> Bit Concat/2
  Bit Slice/1 -> Bit Concat/1
  Bit Slice2/1 -> Bit Concat/3
  Bit Slice3/1 -> Bit Concat/4
  Bit Concat/1 -> out/1

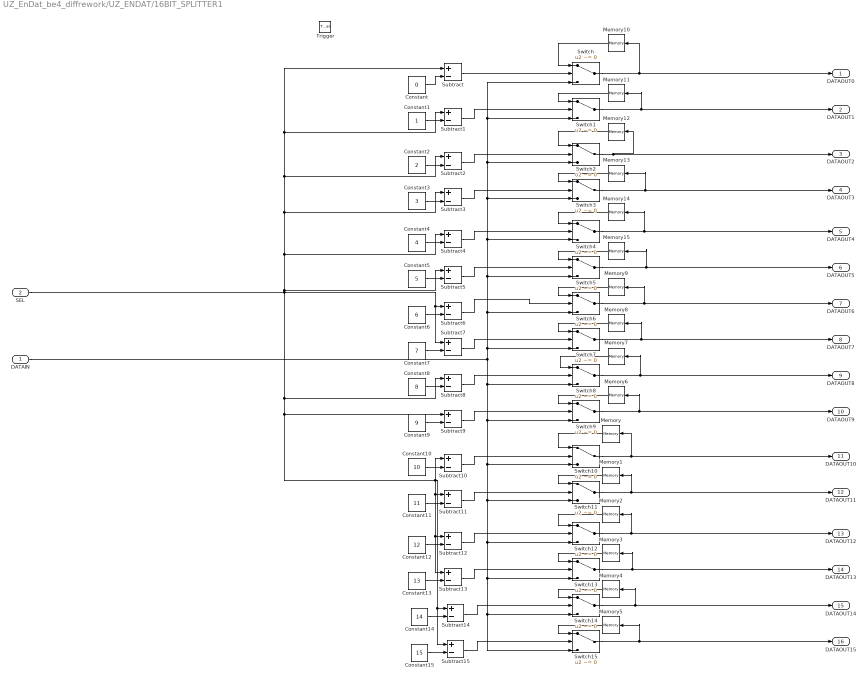
== system UZ_EnDat_be4_diffrework/UZ_ENDAT/16BIT_SPLITTER1 ==
  DATAIN : Inport
  SEL : Inport  Port=2  OutDataTypeStr=fixdt(0,4,0)
  Trigger : TriggerPort  TriggerType=falling  VariantControl=(inherit)  OutputDataType=int8  InitialTriggerSignalState=positive
  Constant : Constant  Value=0  OutDataTypeStr=fixdt(0,4,0)  SampleTime=-1
  Constant1 : Constant  OutDataTypeStr=fixdt(0,4,0)  SampleTime=-1
  Constant10 : Constant  Value=10  OutDataTypeStr=fixdt(0,4,0)  SampleTime=-1
  Constant11 : Constant  Value=11  OutDataTypeStr=fixdt(0,4,0)  SampleTime=-1
  Constant12 : Constant  Value=12  OutDataTypeStr=fixdt(0,4,0)  SampleTime=-1
  Constant13 : Constant  Value=13  OutDataTypeStr=fixdt(0,4,0)  SampleTime=-1
  Constant14 : Constant  Value=14  OutDataTypeStr=fixdt(0,4,0)  SampleTime=-1
  Constant15 : Constant  Value=15  OutDataTypeStr=fixdt(0,4,0)  SampleTime=-1
  Constant2 : Constant  Value=2  OutDataTypeStr=fixdt(0,4,0)  SampleTime=-1
  Constant3 : Constant  Value=3  OutDataTypeStr=fixdt(0,4,0)  SampleTime=-1
  Constant4 : Constant  Value=4  OutDataTypeStr=fixdt(0,4,0)  SampleTime=-1
  Constant5 : Constant  Value=5  OutDataTypeStr=fixdt(0,4,0)  SampleTime=-1
  Constant6 : Constant  Value=6  OutDataTypeStr=fixdt(0,4,0)  SampleTime=-1
  Constant7 : Constant  Value=7  OutDataTypeStr=fixdt(0,4,0)  SampleTime=-1
  Constant8 : Constant  Value=8  OutDataTypeStr=fixdt(0,4,0)  SampleTime=-1
  Constant9 : Constant  Value=9  OutDataTypeStr=fixdt(0,4,0)  SampleTime=-1
  Memory{,1..8,10..11} (11 alike) : Memory  InheritSampleTime=on
  Memory{9,12..15} (5 alike) : Memory  InitialCondition=100  InheritSampleTime=on  LinearizeAsDelay=on
  Subtract{,1..9,11..15} (15 alike) : Sum  Inputs=+-  OutDataTypeStr=fixdt(0,4,0)
  Subtract10 : Sum  Inputs=+-  AccumDataTypeStr=fixdt(0,4,0)
  Switch{,1..15} (16 alike) : Switch  Criteria=u2 ~= 0  SaturateOnIntegerOverflow=off  InputSameDT=off
  DATAOUT0 : Outport  InitialOutput=0
  DATAOUT1 : Outport  Port=2  InitialOutput=0
  DATAOUT2 : Outport  Port=3  InitialOutput=0
  DATAOUT3 : Outport  Port=4  InitialOutput=0
  DATAOUT4 : Outport  Port=5  InitialOutput=0
  DATAOUT5 : Outport  Port=6  InitialOutput=0
  DATAOUT6 : Outport  Port=7  InitialOutput=0
  DATAOUT7 : Outport  Port=8  InitialOutput=0
  DATAOUT8 : Outport  Port=9  InitialOutput=0
  DATAOUT9 : Outport  Port=10  InitialOutput=0
  DATAOUT10 : Outport  Port=11  InitialOutput=0
  DATAOUT11 : Outport  Port=12  InitialOutput=0
  DATAOUT12 : Outport  Port=13  InitialOutput=0
  DATAOUT13 : Outport  Port=14  InitialOutput=0
  DATAOUT14 : Outport  Port=15  InitialOutput=0
  DATAOUT15 : Outport  Port=16  InitialOutput=0
  wires:
  Switch/1 -> Memory10/1, DATAOUT0/1
  Switch1/1 -> Memory11/1, DATAOUT1/1
  Switch3/1 -> Memory13/1, DATAOUT3/1
  Switch2/1 -> Memory12/1, DATAOUT2/1
  Switch5/1 -> Memory15/1, DATAOUT5/1
  Switch4/1 -> Memory14/1, DATAOUT4/1
  Switch7/1 -> Memory8/1, DATAOUT7/1
  Switch6/1 -> Memory9/1, DATAOUT6/1
  Switch9/1 -> Memory6/1, DATAOUT9/1
  Switch10/1 -> Memory/1, DATAOUT10/1
  Switch11/1 -> Memory1/1, DATAOUT11/1
  Switch8/1 -> Memory7/1, DATAOUT8/1
  Switch12/1 -> Memory2/1, DATAOUT12/1
  Switch15/1 -> Memory5/1, DATAOUT15/1
  Switch13/1 -> Memory3/1, DATAOUT13/1
  Switch14/1 -> Memory4/1, DATAOUT14/1
  Constant/1 -> Subtract/2
  Subtract/1 -> Switch/2
  Subtract1/1 -> Switch1/2
  Constant1/1 -> Subtract1/2
  Constant2/1 -> Subtract2/2
  Subtract2/1 -> Switch2/2
  Constant3/1 -> Subtract3/2
  Subtract3/1 -> Switch3/2
  Constant4/1 -> Subtract4/2
  Subtract4/1 -> Switch4/2
  Constant5/1 -> Subtract5/2
  Subtract5/1 -> Switch5/2
  Constant6/1 -> Subtract6/2
  Subtract6/1 -> Switch6/2
  Constant7/1 -> Subtract7/2
  Subtract7/1 -> Switch7/2
  Constant8/1 -> Subtract8/2
  Subtract8/1 -> Switch8/2
  Constant9/1 -> Subtract9/2
  Subtract9/1 -> Switch9/2
  Constant10/1 -> Subtract10/2
  Subtract10/1 -> Switch10/2
  Constant11/1 -> Subtract11/2
  Subtract11/1 -> Switch11/2
  Constant12/1 -> Subtract12/2
  Subtract12/1 -> Switch12/2
  Constant13/1 -> Subtract13/2
  Subtract13/1 -> Switch13/2
  Constant14/1 -> Subtract14/2
  Subtract14/1 -> Switch14/2
  Constant15/1 -> Subtract15/2
  SEL/1 -> Subtract15/1, Subtract14/1, Subtract13/1, Subtract12/1, Subtract11/1, Subtract10/1, Subtract9/1, Subtract8/1, Subtract7/1, Subtract6/1, Subtract5/1, Subtract4/1, Subtract3/1, Subtract2/1, Subtract1/1, Subtract/1
  Subtract15/1 -> Switch15/2
  DATAIN/1 -> Switch4/3, Switch3/3, Switch2/3, Switch1/3, Switch/3, Switch5/3, Switch6/3, Switch7/3, Switch9/3, Switch10/3, Switch11/3, Switch12/3, Switch14/3, Switch15/3, Switch13/3, Switch8/3
  Memory/1 -> Switch10/1
  Memory1/1 -> Switch11/1
  Memory2/1 -> Switch12/1
  Memory3/1 -> Switch13/1
  Memory4/1 -> Switch14/1
  Memory5/1 -> Switch15/1
  Memory6/1 -> Switch9/1
  Memory7/1 -> Switch8/1
  Memory8/1 -> Switch7/1
  Memory9/1 -> Switch6/1
  Memory10/1 -> Switch/1
  Memory11/1 -> Switch1/1
  Memory12/1 -> Switch2/1
  Memory13/1 -> Switch3/1
  Memory14/1 -> Switch4/1
  Memory15/1 -> Switch5/1

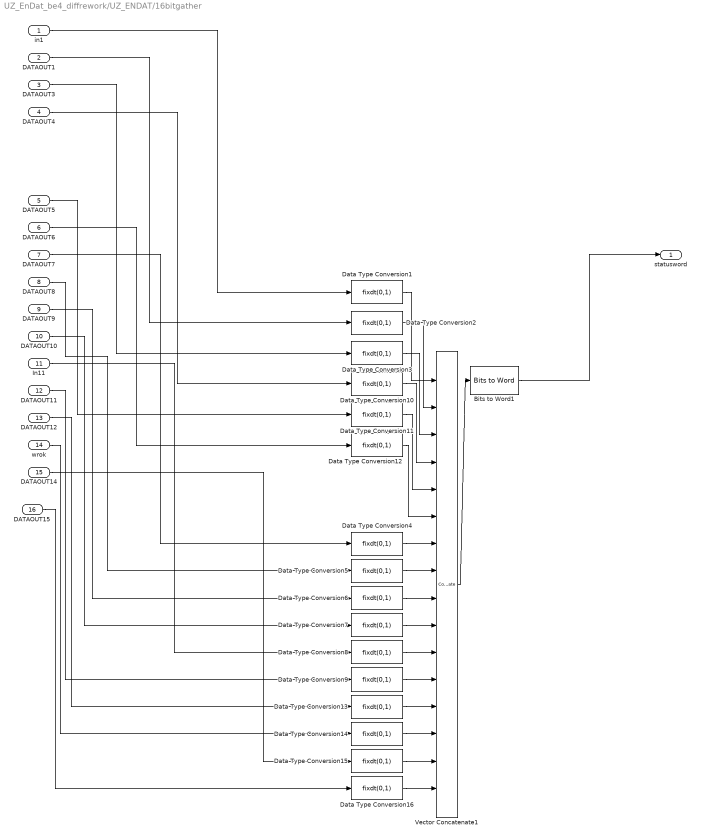
== system UZ_EnDat_be4_diffrework/UZ_ENDAT/16bitgather ==
  in1 : Inport
  DATAOUT1 : Inport  Port=2
  DATAOUT3 : Inport  Port=3
  DATAOUT4 : Inport  Port=4
  DATAOUT5 : Inport  Port=5
  DATAOUT6 : Inport  Port=6
  DATAOUT7 : Inport  Port=7
  DATAOUT8 : Inport  Port=8
  DATAOUT9 : Inport  Port=9
  DATAOUT10 : Inport  Port=10
  In11 : Inport  Port=11
  DATAOUT11 : Inport  Port=12
  DATAOUT12 : Inport  Port=13
  wrok : Inport  Port=14
  DATAOUT14 : Inport  Port=15
  DATAOUT15 : Inport  Port=16
  Bits to Word1 : hdlsllib/Logic and Bit Operations/Bits to Word
  Data Type Conversion{1..16} (16 alike) : DataTypeConversion  OutMax=1  OutDataTypeStr=fixdt(0,1)  SaturateOnIntegerOverflow=off  RndMeth=Floor
  Vector Concatenate1 : Concatenate  NumInputs=16
  statusword : Outport
  wires:
  in1/1 -> Data Type Conversion1/1
  DATAOUT1/1 -> Data Type Conversion2/1
  DATAOUT3/1 -> Data Type Conversion3/1
  DATAOUT4/1 -> Data Type Conversion10/1
  DATAOUT5/1 -> Data Type Conversion11/1
  DATAOUT6/1 -> Data Type Conversion12/1
  DATAOUT7/1 -> Data Type Conversion4/1
  DATAOUT8/1 -> Data Type Conversion5/1
  DATAOUT9/1 -> Data Type Conversion6/1
  DATAOUT10/1 -> Data Type Conversion7/1
  In11/1 -> Data Type Conversion8/1
  DATAOUT11/1 -> Data Type Conversion9/1
  DATAOUT12/1 -> Data Type Conversion13/1
  wrok/1 -> Data Type Conversion14/1
  DATAOUT14/1 -> Data Type Conversion15/1
  Bits to Word1/1 -> statusword/1
  Vector Concatenate1/1 -> Bits to Word1/1
  Data Type Conversion11/1 -> Vector Concatenate1/5
  Data Type Conversion3/1 -> Vector Concatenate1/3
  Data Type Conversion2/1 -> Vector Concatenate1/2
  Data Type Conversion1/1 -> Vector Concatenate1/1
  Data Type Conversion12/1 -> Vector Concatenate1/6
  Data Type Conversion10/1 -> Vector Concatenate1/4
  Data Type Conversion4/1 -> Vector Concatenate1/7
  DATAOUT15/1 -> Data Type Conversion16/1
  Data Type Conversion5/1 -> Vector Concatenate1/8
  Data Type Conversion6/1 -> Vector Concatenate1/9
  Data Type Conversion7/1 -> Vector Concatenate1/10
  Data Type Conversion8/1 -> Vector Concatenate1/11
  Data Type Conversion9/1 -> Vector Concatenate1/12
  Data Type Conversion13/1 -> Vector Concatenate1/13
  Data Type Conversion14/1 -> Vector Concatenate1/14
  Data Type Conversion15/1 -> Vector Concatenate1/15
  Data Type Conversion16/1 -> Vector Concatenate1/16

== system UZ_EnDat_be4_diffrework/UZ_ENDAT/5timestorage ==
  DATA : Inport
  wrok : Inport  Port=2  OutMin=0  OutMax=1  OutDataTypeStr=boolean
  Compare To Constant : hdlsllib/Logic and Bit Operations/Compare To Constant  relop===  const=0  OutDataTypeStr=boolean
  Compare To Constant1 : hdlsllib/Logic and Bit Operations/Compare To Constant  relop===  const=1  OutDataTypeStr=boolean
  Compare To Constant2 : hdlsllib/Logic and Bit Operations/Compare To Constant  relop===  const=2  OutDataTypeStr=boolean
  Compare To Constant3 : hdlsllib/Logic and Bit Operations/Compare To Constant  relop===  const=3  OutDataTypeStr=boolean
  Compare To Constant4 : hdlsllib/Logic and Bit Operations/Compare To Constant  relop===  const=4  OutDataTypeStr=boolean
  Detect Increase{,1..4} (5 alike) : simulink/Logic and Bit Operations/Detect Increase  vinit=0.0  OutDataTypeStr=boolean
      settings: LibrarySourceBlock=|
      | hdlsllib/Logic and Bit
      | Operations/Detect
      | Increase
  Multiport Switch{,1..4} (5 alike) : MultiPortSwitch  DataPortOrder=Zero-based contiguous  Inputs=5  zeroidx=on  SaturateOnIntegerOverflow=off  InputSameDT=off
  Storage1 : Subsystem
      settings: LibrarySourceBlock=|
      | hdlsllib/Ports &
      | Subsystems/Subsystem
  Storage2 : Subsystem
      settings: LibrarySourceBlock=|
      | hdlsllib/Ports &
      | Subsystems/Subsystem
  Storage20 : Subsystem
      settings: LibrarySourceBlock=|
      | hdlsllib/Ports &
      | Subsystems/Subsystem
  Storage3 : Subsystem
      settings: LibrarySourceBlock=|
      | hdlsllib/Ports &
      | Subsystems/Subsystem
  Storage4 : Subsystem
      settings: LibrarySourceBlock=|
      | hdlsllib/Ports &
      | Subsystems/Subsystem
  Triggered Subsystem : Subsystem  TreatAsAtomicUnit=on
      settings: LibrarySourceBlock=|
      | hdlsllib/Ports &
      | Subsystems/Triggered
      | Subsystem
  t0 : Outport
  t-1 : Outport  Port=2
  t-2 : Outport  Port=3
  t-3 : Outport  Port=4
  t-4 : Outport  Port=5  OutDataTypeStr=uint64
  wires:
  Triggered Subsystem/1(Out1) -> Compare To Constant4/1, Compare To Constant3/1, Multiport Switch1/1, Multiport Switch4/1, Multiport Switch3/1, Multiport Switch2/1, Multiport Switch/1, Compare To Constant/1, Compare To Constant1/1, Compare To Constant2/1
  wrok/1 -> Triggered Subsystem/Trigger
  DATA/1 -> Storage4/1(Data), Storage3/1(Data), Storage2/1(Data), Storage1/1(Data), Storage20/1(Data)
  Compare To Constant/1 -> Detect Increase4/1
  Compare To Constant1/1 -> Detect Increase3/1
  Compare To Constant2/1 -> Detect Increase2/1
  Compare To Constant3/1 -> Detect Increase1/1
  Compare To Constant4/1 -> Detect Increase/1
  Storage20/1(out) -> Multiport Switch3/5, Multiport Switch2/4, Multiport Switch/2, Multiport Switch1/3, Multiport Switch4/6
  Storage1/1(out) -> Multiport Switch4/2, Multiport Switch3/6, Multiport Switch2/5, Multiport Switch/3, Multiport Switch1/4
  Multiport Switch/1 -> t0/1
  Storage2/1(out) -> Multiport Switch1/5, Multiport Switch/4, Multiport Switch4/3, Multiport Switch3/2, Multiport Switch2/6
  Storage3/1(out) -> Multiport Switch4/4, Multiport Switch3/3, Multiport Switch2/2, Multiport Switch1/6, Multiport Switch/5
  Storage4/1(out) -> Multiport Switch4/5, Multiport Switch3/4, Multiport Switch2/3, Multiport Switch1/2, Multiport Switch/6
  Multiport Switch1/1 -> t-1/1
  Multiport Switch2/1 -> t-2/1
  Multiport Switch3/1 -> t-3/1
  Multiport Switch4/1 -> t-4/1
  Detect Increase/1 -> Storage4/2(Write)
  Detect Increase1/1 -> Storage3/2(Write)
  Detect Increase2/1 -> Storage2/2(Write)
  Detect Increase3/1 -> Storage1/2(Write)
  Detect Increase4/1 -> Storage20/2(Write)

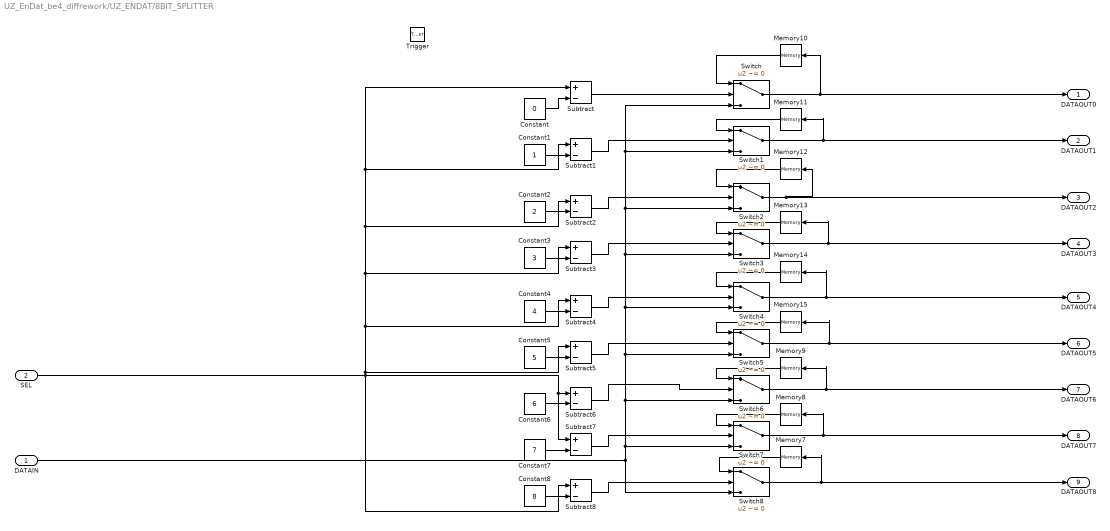
== system UZ_EnDat_be4_diffrework/UZ_ENDAT/8BIT_SPLITTER ==
  DATAIN : Inport
  SEL : Inport  Port=2  OutDataTypeStr=fixdt(0,4,0)
  Trigger : TriggerPort  TriggerType=falling  VariantControl=(inherit)  OutputDataType=int8  InitialTriggerSignalState=positive
  Constant : Constant  Value=0  OutDataTypeStr=fixdt(0,4,0)  SampleTime=-1
  Constant1 : Constant  OutDataTypeStr=fixdt(0,4,0)  SampleTime=-1
  Constant2 : Constant  Value=2  OutDataTypeStr=fixdt(0,4,0)  SampleTime=-1
  Constant3 : Constant  Value=3  OutDataTypeStr=fixdt(0,4,0)  SampleTime=-1
  Constant4 : Constant  Value=4  OutDataTypeStr=fixdt(0,4,0)  SampleTime=-1
  Constant5 : Constant  Value=5  OutDataTypeStr=fixdt(0,4,0)  SampleTime=-1
  Constant6 : Constant  Value=6  OutDataTypeStr=fixdt(0,4,0)  SampleTime=-1
  Constant7 : Constant  Value=7  OutDataTypeStr=fixdt(0,4,0)  SampleTime=-1
  Constant8 : Constant  Value=8  OutDataTypeStr=fixdt(0,4,0)  SampleTime=-1
  Memory{7..8,10..11} (4 alike) : Memory  InheritSampleTime=on
  Memory{9,12..15} (5 alike) : Memory  InitialCondition=100  InheritSampleTime=on  LinearizeAsDelay=on
  Subtract{,1..8} (9 alike) : Sum  Inputs=+-  OutDataTypeStr=fixdt(0,4,0)
  Switch{,1..8} (9 alike) : Switch  Criteria=u2 ~= 0  SaturateOnIntegerOverflow=off  InputSameDT=off
  DATAOUT0 : Outport  InitialOutput=0
  DATAOUT1 : Outport  Port=2  InitialOutput=0
  DATAOUT2 : Outport  Port=3  InitialOutput=0
  DATAOUT3 : Outport  Port=4  InitialOutput=0
  DATAOUT4 : Outport  Port=5  InitialOutput=0
  DATAOUT5 : Outport  Port=6  InitialOutput=0
  DATAOUT6 : Outport  Port=7  InitialOutput=0
  DATAOUT7 : Outport  Port=8  InitialOutput=0
  DATAOUT8 : Outport  Port=9  InitialOutput=0
  wires:
  Switch/1 -> Memory10/1, DATAOUT0/1
  Switch1/1 -> Memory11/1, DATAOUT1/1
  Switch3/1 -> Memory13/1, DATAOUT3/1
  Switch2/1 -> Memory12/1, DATAOUT2/1
  Switch5/1 -> Memory15/1, DATAOUT5/1
  Switch4/1 -> Memory14/1, DATAOUT4/1
  Switch7/1 -> Memory8/1, DATAOUT7/1
  Switch6/1 -> Memory9/1, DATAOUT6/1
  Switch8/1 -> Memory7/1, DATAOUT8/1
  Constant/1 -> Subtract/2
  Subtract/1 -> Switch/2
  Subtract1/1 -> Switch1/2
  Constant1/1 -> Subtract1/2
  Constant2/1 -> Subtract2/2
  Subtract2/1 -> Switch2/2
  Constant3/1 -> Subtract3/2
  Subtract3/1 -> Switch3/2
  Constant4/1 -> Subtract4/2
  Subtract4/1 -> Switch4/2
  Constant5/1 -> Subtract5/2
  Subtract5/1 -> Switch5/2
  Constant6/1 -> Subtract6/2
  Subtract6/1 -> Switch6/2
  Constant7/1 -> Subtract7/2
  Subtract7/1 -> Switch7/2
  Constant8/1 -> Subtract8/2
  Subtract8/1 -> Switch8/2
  ? -> ?
  SEL/1 -> Subtract8/1, Subtract7/1, Subtract6/1, Subtract5/1, Subtract4/1, Subtract3/1, Subtract2/1, Subtract1/1, Subtract/1
  DATAIN/1 -> Switch4/3, Switch3/3, Switch2/3, Switch1/3, Switch/3, Switch5/3, Switch6/3, Switch7/3, Switch8/3
  Memory7/1 -> Switch8/1
  Memory8/1 -> Switch7/1
  Memory9/1 -> Switch6/1
  Memory10/1 -> Switch/1
  Memory11/1 -> Switch1/1
  Memory12/1 -> Switch2/1
  Memory13/1 -> Switch3/1
  Memory14/1 -> Switch4/1
  Memory15/1 -> Switch5/1

== system UZ_EnDat_be4_diffrework/UZ_ENDAT/8BIT_SPLITTER1 ==
  DATAT0 : Inport
  DATAT1 : Inport  Port=2
  DATAT2 : Inport  Port=3
  DATAT3 : Inport  Port=4
  DATAT4 : Inport  Port=5
  Trigger : TriggerPort  TriggerType=falling  VariantControl=(inherit)  OutputDataType=int8  InitialTriggerSignalState=positive
  Subtract{,1..3} (4 alike) : Sum  Inputs=+-  OutDataTypeStr=int32  AccumDataTypeStr=int32  RndMeth=Simplest  SaturateOnIntegerOverflow=on
  DIFT1T0 : Outport  InitialOutput=0
  DIFT2T0 : Outport  Port=2  InitialOutput=0
  DIFT3T0 : Outport  Port=3  InitialOutput=0
  DIFT4T0 : Outport  Port=4  InitialOutput=0
  wires:
  ? -> ?
  DATAT1/1 -> Subtract/2
  DATAT0/1 -> Subtract/1, Subtract1/1, Subtract3/1, Subtract2/1
  Subtract/1 -> DIFT1T0/1
  Subtract1/1 -> DIFT2T0/1
  DATAT2/1 -> Subtract1/2
  DATAT3/1 -> Subtract2/2
  Subtract2/1 -> DIFT3T0/1
  DATAT4/1 -> Subtract3/2
  Subtract3/1 -> DIFT4T0/1

== system UZ_EnDat_be4_diffrework/UZ_ENDAT/CLKCNTER_ACT ==
  CLK : Inport
  CLK2CNT : Inport  Port=2
  ResetCNT : Inport  Port=3  OutDataTypeStr=boolean
  Delay1 : Delay  DelayLength=1
  Positional_Counter : Subsystem  TreatAsAtomicUnit=on
      settings: LibrarySourceBlock=|
      | hdlsllib/Ports &
      | Subsystems/Triggered
      | Subsystem
  SetZero32modified : Subsystem
  CNT : Outport
  wires:
  CLK2CNT/1 -> Positional_Counter/Trigger
  Delay1/1 -> Positional_Counter/1(valueout), CNT/1
  SetZero32modified/1(valueout) -> Delay1/1
  CLK/1 -> SetZero32modified/Trigger
  Positional_Counter/1(divider) -> SetZero32modified/1(valin)
  ResetCNT/1 -> SetZero32modified/2(setzero)
